simulink model "Cantilever Arm model"  (R2016b)
settings: Solver=ode5  StartTime=0.0  StopTime=inf  FixedStep=0.001  RelTol=1e-3  EnableMultiTasking=on
undefined symbols (not defined in the file): Model_626, Sensoray
libraries: sldrtlib x4, simulink x1, powerlib_meascontrol x1
settings Model: SimulationMode=external  Creator=gsmalhi  LastModifiedBy=ferry
settings DataIOCC: LimitDataPoints=on  SaveFormat=Array
settings DebuggingCC: SolverPrmCheckMsg=warning  SFUnexpectedBacktrackingDiag=warning  SFNoUnconditionalDefaultTransitionDiag=warning  SFExecutionAtInitializationDiag=none
settings ModelReferenceCC: PropagateSignalLabelsOutOfModel=off
settings RTWCC: SystemTargetFile=sldrt.tlc  TemplateMakefile=sldrt.tmf  Description=Simulink Desktop Real-Time  RTWCompilerOptimization=on
settings CodeAppCC: MaxIdLength=95
settings SimulinkDesktopRealTimeCC: TargetPreCompLibLocation=C:\Program Files\MATLAB\R2016b\toolbox\sldrt\lib\win64  TargetLangStandard=C89/C90 (ANSI)  SupportVariableSizeSignals=off
settings ConfigComp: CovMetricSettings=dw  CovHtmlReporting=on  CovSaveCumulativeToWorkspaceVar=on  CovSaveSingleToWorkspaceVar=on  CovExternalEMLEnable=off  CovSFcnEnable=off

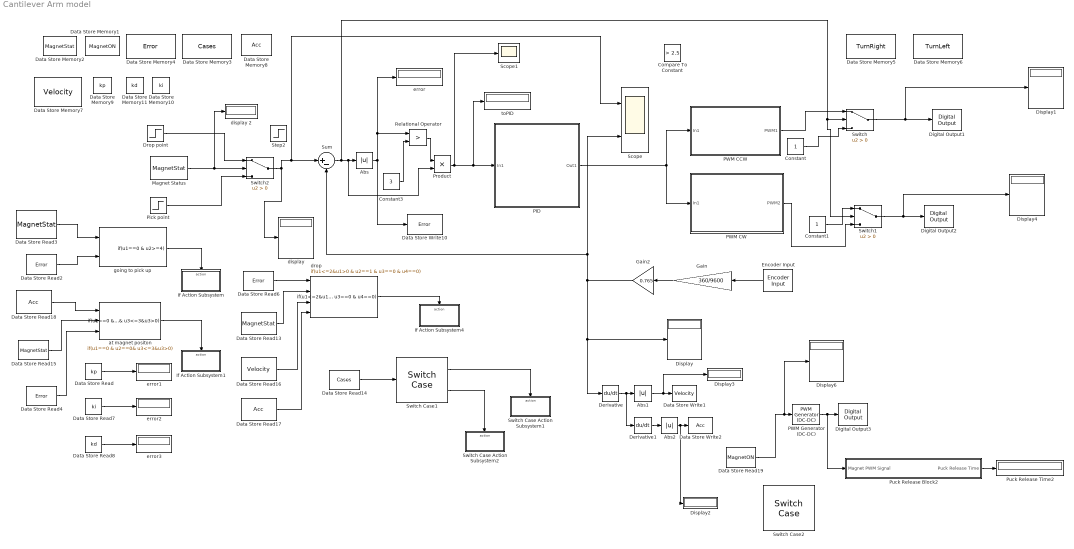
== system Cantilever Arm model ==
  Abs : Abs
  Abs1 : Abs
  Abs2 : Abs
  Compare To Constant : simulink/Logic and Bit Operations/Compare To Constant  relop=>  const=2.5  OutDataTypeStr=uint8
  Constant : Constant
  Constant1 : Constant
  Constant3 : Constant  Value=3  OutDataTypeStr=double
  Data Store Memory1 : DataStoreMemory  DataStoreName=MagnetON  ReadBeforeWriteMsg=warning  WriteAfterWriteMsg=warning  WriteAfterReadMsg=warning  ShowAdditionalParam=off  OutDataTypeStr=double
  Data Store Memory10 : DataStoreMemory  DataStoreName=ki  ReadBeforeWriteMsg=warning  WriteAfterWriteMsg=warning  WriteAfterReadMsg=warning  ShowAdditionalParam=off
  Data Store Memory11 : DataStoreMemory  DataStoreName=kd  ReadBeforeWriteMsg=warning  WriteAfterWriteMsg=warning  WriteAfterReadMsg=warning  ShowAdditionalParam=off
  Data Store Memory2 : DataStoreMemory  DataStoreName=MagnetStat  ReadBeforeWriteMsg=warning  WriteAfterWriteMsg=warning  WriteAfterReadMsg=warning  ShowAdditionalParam=off
  Data Store Memory3 : DataStoreMemory  DataStoreName=Cases  ReadBeforeWriteMsg=warning  WriteAfterWriteMsg=warning  WriteAfterReadMsg=warning  ShowAdditionalParam=off
  Data Store Memory4 : DataStoreMemory  DataStoreName=Error  ReadBeforeWriteMsg=warning  WriteAfterWriteMsg=warning  WriteAfterReadMsg=warning  ShowAdditionalParam=off
  Data Store Memory5 : DataStoreMemory  DataStoreName=TurnRight  ReadBeforeWriteMsg=warning  WriteAfterWriteMsg=warning  WriteAfterReadMsg=warning  ShowAdditionalParam=off
  Data Store Memory6 : DataStoreMemory  DataStoreName=TurnLeft  ReadBeforeWriteMsg=warning  WriteAfterWriteMsg=warning  WriteAfterReadMsg=warning  ShowAdditionalParam=off
  Data Store Memory7 : DataStoreMemory  DataStoreName=Velocity  ReadBeforeWriteMsg=warning  WriteAfterWriteMsg=warning  WriteAfterReadMsg=warning  ShowAdditionalParam=off  OutDataTypeStr=double
  Data Store Memory8 : DataStoreMemory  DataStoreName=Acc  ReadBeforeWriteMsg=warning  WriteAfterWriteMsg=warning  WriteAfterReadMsg=warning  ShowAdditionalParam=off  OutDataTypeStr=double
  Data Store Memory9 : DataStoreMemory  DataStoreName=kp  ReadBeforeWriteMsg=warning  WriteAfterWriteMsg=warning  WriteAfterReadMsg=warning  ShowAdditionalParam=off
  Data Store Read : DataStoreRead  DataStoreName=kp
  Data Store Read13 : DataStoreRead  DataStoreName=MagnetStat
  Data Store Read14 : DataStoreRead  DataStoreName=Cases
  Data Store Read15 : DataStoreRead  DataStoreName=MagnetStat
  Data Store Read16 : DataStoreRead  DataStoreName=Velocity
  Data Store Read17 : DataStoreRead  DataStoreName=Acc
  Data Store Read18 : DataStoreRead  DataStoreName=Acc
  Data Store Read19 : DataStoreRead  DataStoreName=MagnetON
  Data Store Read2 : DataStoreRead  DataStoreName=Error
  Data Store Read3 : DataStoreRead  DataStoreName=MagnetStat
  Data Store Read4 : DataStoreRead  DataStoreName=Error
  Data Store Read6 : DataStoreRead  DataStoreName=Error
  Data Store Read7 : DataStoreRead  DataStoreName=ki
  Data Store Read8 : DataStoreRead  DataStoreName=kd
  Data Store Write1 : DataStoreWrite  DataStoreName=Velocity
  Data Store Write10 : DataStoreWrite  DataStoreName=Error
  Data Store Write2 : DataStoreWrite  DataStoreName=Acc
  Derivative : Derivative
  Derivative1 : Derivative
  Digital Output1 : sldrtlib/Digital Output  SampleTime=0.001  MaxMissedTicks=10  ShowMissedTicks=off  YieldWhenWaiting=off  DrvName=Sensoray/Model_626  DrvAddress=4294967295  DrvOptions=zeros(1,0)  Channels=1  BitMode=1  InitialValue=[]  FinalValue=[]
      settings: AttributesFormatString=Sensoray\nModel 626 [auto]
  Digital Output2 : sldrtlib/Digital Output  SampleTime=0.001  MaxMissedTicks=10  ShowMissedTicks=off  YieldWhenWaiting=off  DrvName=Sensoray/Model_626  DrvAddress=4294967295  DrvOptions=zeros(1,0)  Channels=2  BitMode=1  InitialValue=[]  FinalValue=[]
      settings: AttributesFormatString=Sensoray\nModel 626 [auto]
  Digital Output3 : sldrtlib/Digital Output  SampleTime=0.001  MaxMissedTicks=10  ShowMissedTicks=off  YieldWhenWaiting=off  DrvName=Sensoray/Model_626  DrvAddress=4294967295  DrvOptions=zeros(1,0)  Channels=3  BitMode=1  InitialValue=[]  FinalValue=[]
      settings: AttributesFormatString=Sensoray\nModel 626 [auto]
  Display{,1..4,6} (6 alike) : Display
  "Drop point " : Step  Time=0  After=135  SampleTime=0
  Encoder Input : sldrtlib/Encoder Input  SampleTime=0.001  MaxMissedTicks=10  ShowMissedTicks=off  YieldWhenWaiting=off  DrvName=Sensoray/Model_626  DrvAddress=4294967295  DrvOptions=zeros(1,0)  Channels=[1]  QuadMode=3  IndexPulse=2  InputFilter=Inf  DataType=1
      settings: AttributesFormatString=Sensoray\nModel 626 [auto]
  Gain : Gain  Gain=360/9600
  Gain2 : Gain  Gain=0.765
  If Action Subsystem : Subsystem  TreatAsAtomicUnit=on
  If Action Subsystem1 : Subsystem  TreatAsAtomicUnit=on
  If Action Subsystem4 : Subsystem  TreatAsAtomicUnit=on
  Magnet Status : DataStoreRead  DataStoreName=MagnetStat
  PID : Subsystem
  PWM CCW : Subsystem
  PWM CW : Subsystem
  PWM Generator (DC-DC) : powerlib_meascontrol/Pulse & Signal Generators/PWM Generator (DC-DC)  Fsw=100  Ts=.001
  Pick point : Step  Time=0  After=-45  SampleTime=0
  Product : Product
  Puck Release Block2 : Subsystem
  Puck Release Time2 : Display
  Relational Operator : RelationalOperator  Operator=>  RndMeth=Nearest
  Scope : Scope  NumInputPorts=2
  Scope1 : Scope
  Step2 : Step  After=-45  SampleTime=0
  Sum : Sum  Inputs=|+-
  Switch : Switch  Criteria=u2 > Threshold
  Switch Case Action Subsystem1 : Subsystem  TreatAsAtomicUnit=on
  Switch Case Action Subsystem2 : Subsystem  TreatAsAtomicUnit=on
  Switch Case1 : SwitchCase  CaseConditions={1,[2]}  ShowDefaultCase=off
  Switch Case2 : SwitchCase  CaseConditions={1,[2]}
  Switch1 : Switch  Criteria=u2 > Threshold
  Switch2 : Switch  Criteria=u2 > Threshold
  "at magnet positon " : If  NumInputs=3  IfExpression=u1==0 & u2==0& u3<=3&u3>0  ShowElse=off
  "display " : Display
  display 2 : Display
  drop : If  NumInputs=4  IfExpression=u1<=2&u1>0 & u2==1 & u3==0 & u4==0  ShowElse=off
  error{,1..3} (4 alike) : Display
  "going to pick up " : If  NumInputs=2  IfExpression=u1==0 & u2>=4  ShowElse=off
  toPID : Display
  wires:
  Encoder Input/1 -> Gain/1
  Gain/1 -> Gain2/1
  PWM CW/1(PWM2) -> Switch1/3
  Sum/1 -> Abs/1, Product/2, Switch1/2, Switch/2
  Product/1 -> toPID/1, PID/1(In1), Scope1/1
  PID/1(Out1) -> PWM CW/1(In1), PWM CCW/1(In1)
  PWM CCW/1(PWM1) -> Switch/1
  Constant/1 -> Switch/3
  Constant1/1 -> Switch1/1
  Gain2/1 -> Derivative/1, Display/1, Scope/2, Sum/2
  Abs/1 -> Relational Operator/1, error/1, Data Store Write10/1
  PWM Generator (DC-DC)/1 -> Puck Release Block2/1(Magnet PWM Signal), Digital Output3/1
  Switch/1 -> Digital Output1/1, Display1/1
  Switch1/1 -> Digital Output2/1, Display4/1
  Magnet Status/1 -> display 2/1, Switch2/2
  Pick point/1 -> Switch2/3
  Data Store Read2/1 -> "going to pick up "/2
  Data Store Read3/1 -> "going to pick up "/1
  "going to pick up "/1 -> If Action Subsystem/Action
  "at magnet positon "/1 -> If Action Subsystem1/Action
  Switch2/1 -> Sum/1, Scope/1, "display "/1
  Data Store Read7/1 -> error2/1
  Data Store Read/1 -> error1/1
  Data Store Read8/1 -> error3/1
  "Drop point "/1 -> Switch2/1
  Derivative/1 -> Derivative1/1, Abs1/1
  Abs1/1 -> Display3/1, Data Store Write1/1
  Data Store Read6/1 -> drop/1
  Data Store Read13/1 -> drop/2
  drop/1 -> If Action Subsystem4/Action
  Switch Case1/1 -> Switch Case Action Subsystem1/Action
  Derivative1/1 -> Abs2/1
  Abs2/1 -> Display2/1, Data Store Write2/1
  Data Store Read14/1 -> Switch Case1/1
  Data Store Read15/1 -> "at magnet positon "/2
  Switch Case1/2 -> Switch Case Action Subsystem2/Action
  Data Store Read16/1 -> drop/3
  Data Store Read17/1 -> drop/4
  Data Store Read19/1 -> Display6/1, PWM Generator (DC-DC)/1
  Data Store Read18/1 -> "at magnet positon "/1
  Data Store Read4/1 -> "at magnet positon "/3
  Relational Operator/1 -> Product/1
  Constant3/1 -> Relational Operator/2
  Puck Release Block2/1(Puck Release Time) -> Puck Release Time2/1

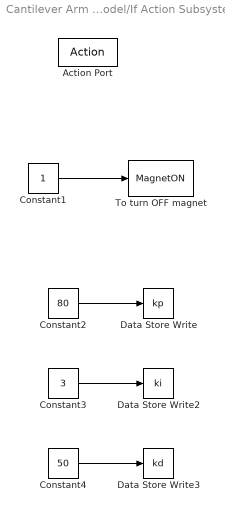
== system Cantilever Arm model/If Action Subsystem ==
  Action Port : ActionPort  ActionType=then
  Constant1 : Constant
  Constant2 : Constant  Value=80
  Constant3 : Constant  Value=3
  Constant4 : Constant  Value=50
  Data Store Write : DataStoreWrite  DataStoreName=kp  DataStoreElements=kp
  Data Store Write2 : DataStoreWrite  DataStoreName=ki
  Data Store Write3 : DataStoreWrite  DataStoreName=kd
  To turn OFF magnet : DataStoreWrite  DataStoreName=MagnetON
  wires:
  Constant1/1 -> To turn OFF magnet/1
  Constant2/1 -> Data Store Write/1
  Constant4/1 -> Data Store Write3/1
  Constant3/1 -> Data Store Write2/1

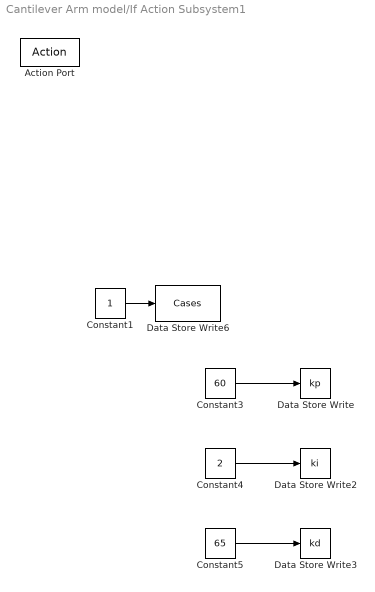
== system Cantilever Arm model/If Action Subsystem1 ==
  Action Port : ActionPort  ActionType=then
  Constant1 : Constant
  Constant3 : Constant  Value=60
  Constant4 : Constant  Value=2
  Constant5 : Constant  Value=65
  Data Store Write : DataStoreWrite  DataStoreName=kp  DataStoreElements=kp
  Data Store Write2 : DataStoreWrite  DataStoreName=ki
  Data Store Write3 : DataStoreWrite  DataStoreName=kd
  Data Store Write6 : DataStoreWrite  DataStoreName=Cases
  wires:
  Constant3/1 -> Data Store Write/1
  Constant5/1 -> Data Store Write3/1
  Constant4/1 -> Data Store Write2/1
  Constant1/1 -> Data Store Write6/1

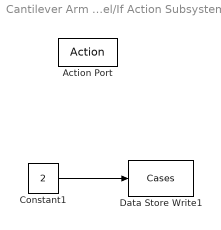
== system Cantilever Arm model/If Action Subsystem4 ==
  Action Port : ActionPort  ActionType=then
  Constant1 : Constant  Value=2
  Data Store Write1 : DataStoreWrite  DataStoreName=Cases
  wires:
  Constant1/1 -> Data Store Write1/1

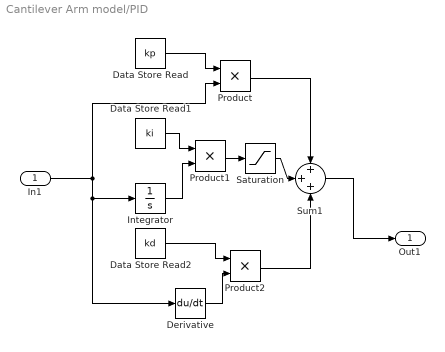
== system Cantilever Arm model/PID ==
  In1 : Inport
  Data Store Read : DataStoreRead  DataStoreName=kp
  Data Store Read1 : DataStoreRead  DataStoreName=ki
  Data Store Read2 : DataStoreRead  DataStoreName=kd
  Derivative : Derivative
  Integrator : Integrator
  Product : Product
  Product1 : Product
  Product2 : Product
  Saturation : Saturate  LowerLimit=0
  Sum1 : Sum  Inputs=+++
  Out1 : Outport
  wires:
  Product/1 -> Sum1/1
  Integrator/1 -> Product1/2
  Derivative/1 -> Product2/2
  Product2/1 -> Sum1/3
  Sum1/1 -> Out1/1
  In1/1 -> Derivative/1, Integrator/1, Product/2
  Data Store Read/1 -> Product/1
  Data Store Read1/1 -> Product1/1
  Data Store Read2/1 -> Product2/1
  Product1/1 -> Saturation/1
  Saturation/1 -> Sum1/2

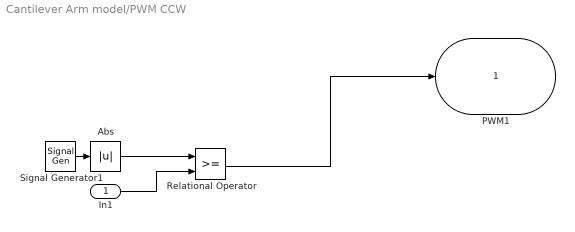
== system Cantilever Arm model/PWM CCW ==
  In1 : Inport
  Abs : Abs
  Relational Operator : RelationalOperator  OutDataTypeStr=boolean  RndMeth=Nearest
  Signal Generator1 : SignalGenerator  WaveForm=sawtooth  Amplitude=5  Frequency=100
  PWM1 : Outport
  wires:
  In1/1 -> Relational Operator/2
  Relational Operator/1 -> PWM1/1
  Signal Generator1/1 -> Abs/1
  Abs/1 -> Relational Operator/1

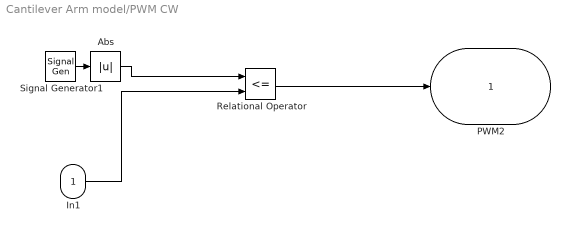
== system Cantilever Arm model/PWM CW ==
  In1 : Inport
  Abs : Abs
  Relational Operator : RelationalOperator  Operator=<=  OutDataTypeStr=boolean  RndMeth=Nearest
  Signal Generator1 : SignalGenerator  WaveForm=sawtooth  Amplitude=5  Frequency=100
  PWM2 : Outport
  wires:
  Relational Operator/1 -> PWM2/1
  In1/1 -> Relational Operator/2
  Signal Generator1/1 -> Abs/1
  Abs/1 -> Relational Operator/1

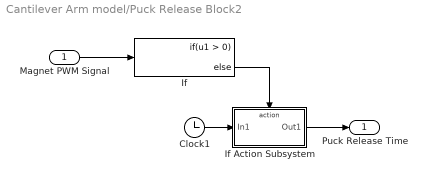
== system Cantilever Arm model/Puck Release Block2 ==
  Magnet PWM Signal : Inport
  Clock1 : Clock
  If : If
  If Action Subsystem : Subsystem  TreatAsAtomicUnit=on
  Puck Release Time : Outport
  wires:
  Clock1/1 -> If Action Subsystem/1(In1)
  Magnet PWM Signal/1 -> If/1
  If Action Subsystem/1(Out1) -> Puck Release Time/1
  If/2 -> If Action Subsystem/Action

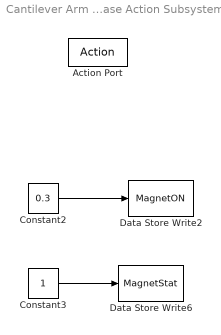
== system Cantilever Arm model/Switch Case Action Subsystem1 ==
  Action Port : ActionPort  ActionType=case
  Constant2 : Constant  Value=0.3  OutDataTypeStr=double
  Constant3 : Constant
  Data Store Write2 : DataStoreWrite  DataStoreName=MagnetON
  Data Store Write6 : DataStoreWrite  DataStoreName=MagnetStat
  wires:
  Constant2/1 -> Data Store Write2/1
  Constant3/1 -> Data Store Write6/1

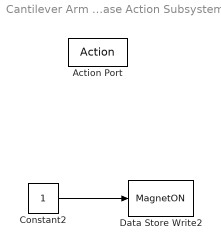
== system Cantilever Arm model/Switch Case Action Subsystem2 ==
  Action Port : ActionPort  ActionType=case
  Constant2 : Constant
  Data Store Write2 : DataStoreWrite  DataStoreName=MagnetON
  wires:
  Constant2/1 -> Data Store Write2/1

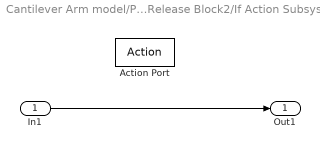
== system Cantilever Arm model/Puck Release Block2/If Action Subsystem ==
  In1 : Inport
  Action Port : ActionPort  ActionType=else
  Out1 : Outport
  wires:
  In1/1 -> Out1/1
